simulink model "SC228_TrackedRadarModelUnitTest"  (R2018b)
settings: Solver=VariableStepAuto  StartTime=0.0  StopTime=180  RelTol=1e-3
model workspace (MAT data in the model file):
  MCOS : class17 (value not decoded)
  MCOS : class17 (value not decoded)
  MCOS : class17 (value not decoded)
  MCOS : class17 (value not decoded)
  MCOS : class17 (value not decoded)
  MCOS : class17 (value not decoded)
  N_tracked_random_stddev_ft = 250
  MCOS : class17 (value not decoded)
  MCOS : class17 (value not decoded)
  MCOS : class17 (value not decoded)
  MCOS : class17 (value not decoded)
  MCOS : class17 (value not decoded)
  MCOS : class17 (value not decoded)
  MCOS : class17 (value not decoded)
undefined symbols (not defined in the file or in its folder): ac1dyn_alt0_ft, ac1dyn_con, ac1dyn_lat0_rad, ac1dyn_lon0_rad, ac2dyn_alt0_ft, ac2dyn_con, ac2dyn_lat0_rad, ac2dyn_lon0_rad, ddh_ftps2, dh_ftps, dv_ftps2, e_ft, Edot_ftps, h_ft, hdot_ftps, latLonAltState, n_ft, Ndot_ftps, p_radps, phi_rad, phidot_radps, psi_rad, psidot_radps, q_radps, r_radps, theta_rad, thetadot_radps, uas_rdr_trckd_az_bias_ft, uas_rdr_trckd_az_bias_rad, uas_rdr_trckd_az_random_stddev_rad, uas_rdr_trckd_az_stddev_ft, uas_rdr_trckd_azdot_bias_ftps, uas_rdr_trckd_azdot_stddev_ftps, uas_rdr_trckd_debugMode, uas_rdr_trckd_dt_s, uas_rdr_trckd_el_bias_ft, uas_rdr_trckd_el_bias_rad, uas_rdr_trckd_el_random_stddev_rad, uas_rdr_trckd_el_stddev_ft, uas_rdr_trckd_eldot_bias_ftps, uas_rdr_trckd_eldot_stddev_ftps, uas_rdr_trckd_RCPR_Mode, uas_rdr_trckd_RCPR_Range_ft, uas_rdr_trckd_reported_errorCovRAE, uas_rdr_trckd_rng_bias_ft, uas_rdr_trckd_rng_random_stddev_ft, uas_rdr_trckd_rngdot_bias_ftps, uas_rdr_trckd_rngdot_random_stddev_ftps, uas_rdr_trckd_seed1, uas_rdr_trckd_seed2, uas_rdr_trckd_seed3, uas_rdr_trckd_seed4, uas_rdr_trckd_sns_for_azimuth_deg, uas_rdr_trckd_sns_for_elevation_deg, v_ftps, vdot_fpss
libraries: simulink x17, dspmtrx3 x1
(part 2 of 2)

== system SC228_TrackedRadarModelUnitTest/AC2 - Track Following/Follow Trajectory/Compute Euler Angles ==
  AircraftState : Inport
  Constraints : Inport  Port=2
  Bus Selector : BusSelector  OutputSignals=psi_rad,theta_rad,phi_rad
  Bus Selector1 : BusSelector  OutputSignals=dphi_radps_max
  Discrete Derivative : simulink/Discrete/Discrete Derivative  gainval=1.0  ICPrevScaledInput=0.0  OutMin=[]  OutMax=[]  OutDataType=fixdt(1, 16)  OutScaling=2^-10  DoSatur=off
  Discrete Derivative1 : simulink/Discrete/Discrete Derivative  gainval=1.0  ICPrevScaledInput=0.0  OutMin=[]  OutMax=[]  OutDataType=fixdt(1, 16)  OutScaling=2^-10  DoSatur=off
  Discrete Derivative2 : simulink/Discrete/Discrete Derivative  gainval=1.0  ICPrevScaledInput=0.0  OutMin=[]  OutMax=[]  OutDataType=fixdt(1, 16)  OutScaling=2^-10  DoSatur=off
  IC : InitialCondition  Value=0
  IC1 : InitialCondition  Value=0
  IC2 : InitialCondition  Value=0
  Saturation Dynamic : simulink/Discontinuities/Saturation Dynamic  OutMin=[]  OutMax=[]  OutDataTypeStr=Inherit: Same as second input  OutDataType=fixdt(1, 16)  OutScaling=2^-10  DoSatur=off
  Unary Minus : UnaryMinus
  Psi Dot : Outport
  Theta Dot : Outport  Port=2
  "Phi Dot " : Outport  Port=3
  wires:
  Constraints/1 -> Bus Selector1/1
  IC2/1 -> Saturation Dynamic/2
  IC1/1 -> Theta Dot/1
  IC/1 -> Psi Dot/1
  Discrete Derivative2/1 -> IC2/1
  Discrete Derivative1/1 -> IC1/1
  Discrete Derivative/1 -> IC/1
  Bus Selector/3 -> Discrete Derivative2/1  "<phi_rad>"
  Bus Selector/2 -> Discrete Derivative1/1  "<theta_rad>"
  Bus Selector/1 -> Discrete Derivative/1  "<psi_rad>"
  AircraftState/1 -> Bus Selector/1
  Saturation Dynamic/1 -> "Phi Dot "/1
  Bus Selector1/1 -> Unary Minus/1, Saturation Dynamic/1  "<dphi_radps_max>"
  Unary Minus/1 -> Saturation Dynamic/3

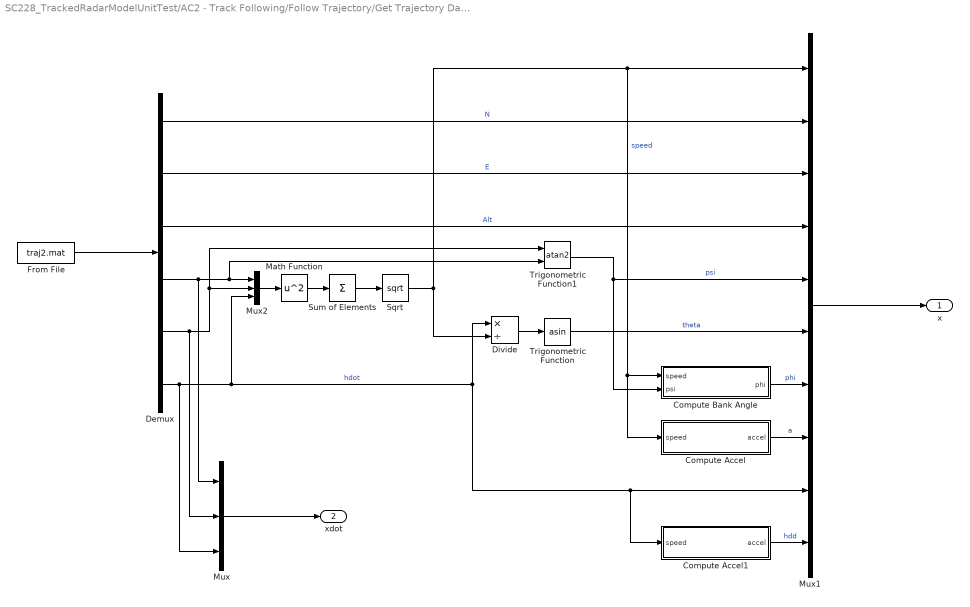
== system SC228_TrackedRadarModelUnitTest/AC2 - Track Following/Follow Trajectory/Get Trajectory Data ==
  Compute Accel : Subsystem
  Compute Accel1 : Subsystem
  Compute Bank Angle : Subsystem
  Demux : Demux  Outputs=6
  Divide : Product  Inputs=*/
  From File : FromFile  FileName=traj2.mat  SampleTime=0.1
  Math Function : Math  Operator=square  SaturateOnIntegerOverflow=on
  Mux : Mux  Inputs=3
  Mux1 : Mux  Inputs=10
  Mux2 : Mux  Inputs=3
  Sqrt : Sqrt  SaturateOnIntegerOverflow=on
  Sum of Elements : Sum  Inputs=+
  Trigonometric Function : Trigonometry  Operator=asin
  Trigonometric Function1 : Trigonometry  Operator=atan2
  x : Outport
  xdot : Outport  Port=2
  wires:
  Mux/1 -> xdot/1
  Compute Accel1/1(accel) -> Mux1/10  "hdd"
  Demux/5 -> Mux2/2, Trigonometric Function1/1, Mux/2
  Divide/1 -> Trigonometric Function/1
  Trigonometric Function1/1 -> Mux1/5, Compute Bank Angle/2(psi)  "psi"
  Trigonometric Function/1 -> Mux1/6  "theta"
  Compute Bank Angle/1(phi) -> Mux1/7  "phi"
  Compute Accel/1(accel) -> Mux1/8  "a"
  Mux1/1 -> x/1
  Sqrt/1 -> Divide/2, Mux1/1, Compute Bank Angle/1(speed), Compute Accel/1(speed)  "speed"
  Sum of Elements/1 -> Sqrt/1
  Math Function/1 -> Sum of Elements/1
  Mux2/1 -> Math Function/1
  Demux/6 -> Mux1/9, Compute Accel1/1(speed), Divide/1, Mux2/3, Mux/3  "hdot"
  Demux/4 -> Mux2/1, Trigonometric Function1/2, Mux/1
  Demux/3 -> Mux1/4  "Alt"
  Demux/2 -> Mux1/3  "E"
  Demux/1 -> Mux1/2  "N"
  From File/1 -> Demux/1

== system SC228_TrackedRadarModelUnitTest/AC2 - Track Following/Follow Trajectory/Null State Rate ==
  Bus Creator : BusCreator  Inputs='vdot_fpss','Ndot_ftps','Edot_ftps','hdot_ftps','psidot_radps','thetadot_radps','phidot_radps'  OutDataTypeStr=Bus: AircraftStateRate
  Constant{,1..6} (7 alike) : Constant  Value=0
  StateRate : Outport  OutDataTypeStr=Bus: AircraftStateRate
  wires:
  Constant6/1 -> Bus Creator/7  "phidot_radps"
  Constant5/1 -> Bus Creator/6  "thetadot_radps"
  Constant4/1 -> Bus Creator/5  "psidot_radps"
  Constant3/1 -> Bus Creator/4  "hdot_ftps"
  Constant2/1 -> Bus Creator/3  "Edot_ftps"
  Constant1/1 -> Bus Creator/2  "Ndot_ftps"
  Constant/1 -> Bus Creator/1  "vdot_fpss"
  Bus Creator/1 -> StateRate/1

== system SC228_TrackedRadarModelUnitTest/AC2 - Track Following/Follow Trajectory/Set LLA  ==
  State In : Inport
  Bus Assignment : BusAssignment  AssignedSignals=latLonAltState.lat_rad,latLonAltState.lon_rad,latLonAltState.dlat_radps,latLonAltState.dlon_radps,latLonAltState.alt_ft,latLonAltState.dalt_ftps
  Bus Selector : BusSelector  OutputSignals=e_ft,n_ft,h_ft,v_ftps,psi_rad,theta_rad
  Constant : Constant  Value=lat0
  Constant7 : Constant  Value=lon0
  Constant8 : Constant  Value=h0
  MATLAB Function : MATLAB Function  TreatAsAtomicUnit=on
  State Out : Outport
  wires:
  Bus Selector/6 -> MATLAB Function/6(theta_rad)  "<theta_rad>"
  Bus Selector/5 -> MATLAB Function/5(psi_rad)  "<psi_rad>"
  Bus Selector/4 -> MATLAB Function/4(v_ftps)  "<v_ftps>"
  Bus Selector/3 -> MATLAB Function/3(u_ft)  "<h_ft>"
  Bus Selector/2 -> MATLAB Function/2(n_ft)  "<n_ft>"
  Bus Selector/1 -> MATLAB Function/1(e_ft)  "<e_ft>"
  Constant8/1 -> MATLAB Function/9(h0)
  Constant7/1 -> MATLAB Function/8(lon0)
  Constant/1 -> MATLAB Function/7(lat0)
  State In/1 -> Bus Selector/1, Bus Assignment/1
  Bus Assignment/1 -> State Out/1
  MATLAB Function/6(dalt_ftps) -> Bus Assignment/7  "dalt_ftps"
  MATLAB Function/5(alt_ft) -> Bus Assignment/6  "alt_ft"
  MATLAB Function/4(dlon_radps) -> Bus Assignment/5  "dlon_radps"
  MATLAB Function/3(dlat_radps) -> Bus Assignment/4  "dlat_radps"
  MATLAB Function/2(lon_rad) -> Bus Assignment/3  "lon_rad"
  MATLAB Function/1(lat_rad) -> Bus Assignment/2  "lat_rad"

== system SC228_TrackedRadarModelUnitTest/AC2 - Track Following/Follow Trajectory/Set State ==
  x : Inport
  Bus Assignment : BusAssignment  AssignedSignals=v_ftps,n_ft,e_ft,h_ft,psi_rad,theta_rad,phi_rad,dv_ftps2,dh_ftps,ddh_ftps2
  Demux : Demux  Outputs=10
  Null AircraftState : Subsystem
  State : Outport
  wires:
  Demux/10 -> Bus Assignment/11
  Demux/9 -> Bus Assignment/10
  Bus Assignment/1 -> State/1
  Null AircraftState/1(State) -> Bus Assignment/1
  Demux/7 -> Bus Assignment/8  "phi"
  x/1 -> Demux/1
  Demux/6 -> Bus Assignment/7  "theta"
  Demux/5 -> Bus Assignment/6  "psi"
  Demux/4 -> Bus Assignment/5  "h"
  Demux/3 -> Bus Assignment/4  "E"
  Demux/2 -> Bus Assignment/3  "N"
  Demux/1 -> Bus Assignment/2  "v"
  Demux/8 -> Bus Assignment/9  "a"

== system SC228_TrackedRadarModelUnitTest/SC-228 Sensor Model: Radar (Tracked)/Add Errors/Colored Noise1 ==
  Add : Sum  Inputs=+++  SampleTime=dt
  Add1 : Sum  SampleTime=dt
  Constant : Constant  Value=false
  Constant1 : Constant  Value=0
  Gain : Gain  Gain=exp(-dt(1)/tau)  SampleTime=dt
  Gain1 : Gain  Gain=sig*sqrt(1-(exp(-dt(1)/tau))*(exp(-dt(1)/tau)))
  Gain2 : Gain  Gain=sig
  IsInitial : Memory  InitialCondition=true  InheritSampleTime=on
  Memory : Memory  InheritSampleTime=on
  Random Number : RandomNumber  Seed=seed  SampleTime=dt_s
  Switch : Switch  Criteria=u2 ~= 0  SampleTime=dt
  bias : Constant  Value=bias
  noisy : Outport
  wires:
  Gain2/1 -> Switch/1
  Add1/1 -> Switch/3  "colored random error"
  IsInitial/1 -> Switch/2
  Constant/1 -> IsInitial/1
  Memory/1 -> Gain/1
  Add/1 -> noisy/1  "noisy state parameter"
  Gain/1 -> Add1/1  "correlated error"
  Random Number/1 -> Gain1/1, Gain2/1
  bias/1 -> Add/2  "fixed bias"
  Switch/1 -> Add/3, Memory/1  "colored random error"
  Gain1/1 -> Add1/2  "uncorrelated error"
  Constant1/1 -> Add/1

== system SC228_TrackedRadarModelUnitTest/SC-228 Sensor Model: Radar (Tracked)/Add Errors/Colored Noise2 ==
  Add : Sum  Inputs=+++  SampleTime=dt
  Add1 : Sum  SampleTime=dt
  Constant : Constant  Value=false
  Constant1 : Constant  Value=0
  Gain : Gain  Gain=exp(-dt(1)/tau)  SampleTime=dt
  Gain1 : Gain  Gain=sig*sqrt(1-(exp(-dt(1)/tau))*(exp(-dt(1)/tau)))
  Gain2 : Gain  Gain=sig
  IsInitial : Memory  InitialCondition=true  InheritSampleTime=on
  Memory : Memory  InheritSampleTime=on
  Random Number : RandomNumber  Seed=seed  SampleTime=dt_s
  Switch : Switch  Criteria=u2 ~= 0  SampleTime=dt
  bias : Constant  Value=0
  noisy : Outport
  wires:
  Gain2/1 -> Switch/1
  Add1/1 -> Switch/3  "colored random error"
  IsInitial/1 -> Switch/2
  Constant/1 -> IsInitial/1
  Memory/1 -> Gain/1
  Add/1 -> noisy/1  "noisy state parameter"
  Gain/1 -> Add1/1  "correlated error"
  Random Number/1 -> Gain1/1, Gain2/1
  bias/1 -> Add/2  "fixed bias"
  Switch/1 -> Add/3, Memory/1  "colored random error"
  Gain1/1 -> Add1/2  "uncorrelated error"
  Constant1/1 -> Add/1

== system SC228_TrackedRadarModelUnitTest/SC-228 Sensor Model: Radar (Tracked)/Add Errors/Colored Noise3 ==
  Add : Sum  Inputs=+++  SampleTime=dt
  Add1 : Sum  SampleTime=dt
  Constant : Constant  Value=false
  Constant1 : Constant  Value=0
  Gain : Gain  Gain=exp(-dt(1)/tau)  SampleTime=dt
  Gain1 : Gain  Gain=sig*sqrt(1-(exp(-dt(1)/tau))*(exp(-dt(1)/tau)))
  Gain2 : Gain  Gain=sig
  IsInitial : Memory  InitialCondition=true  InheritSampleTime=on
  Memory : Memory  InheritSampleTime=on
  Random Number : RandomNumber  Seed=seed  SampleTime=dt_s
  Switch : Switch  Criteria=u2 ~= 0  SampleTime=dt
  bias : Constant  Value=0
  noisy : Outport
  wires:
  Gain2/1 -> Switch/1
  Add1/1 -> Switch/3  "colored random error"
  IsInitial/1 -> Switch/2
  Constant/1 -> IsInitial/1
  Memory/1 -> Gain/1
  Add/1 -> noisy/1  "noisy state parameter"
  Gain/1 -> Add1/1  "correlated error"
  Random Number/1 -> Gain1/1, Gain2/1
  bias/1 -> Add/2  "fixed bias"
  Switch/1 -> Add/3, Memory/1  "colored random error"
  Gain1/1 -> Add1/2  "uncorrelated error"
  Constant1/1 -> Add/1

== system SC228_TrackedRadarModelUnitTest/SC-228 Sensor Model: Radar (Tracked)/Add Errors/Colored Noise4 ==
  Add : Sum  Inputs=+++  SampleTime=dt
  Add1 : Sum  SampleTime=dt
  Constant : Constant  Value=false
  Constant1 : Constant  Value=0
  Gain : Gain  Gain=exp(-dt(1)/tau)  SampleTime=dt
  Gain1 : Gain  Gain=sig*sqrt(1-(exp(-dt(1)/tau))*(exp(-dt(1)/tau)))
  Gain2 : Gain  Gain=sig
  IsInitial : Memory  InitialCondition=true  InheritSampleTime=on
  Memory : Memory  InheritSampleTime=on
  Random Number : RandomNumber  Seed=seed  SampleTime=dt_s
  Switch : Switch  Criteria=u2 ~= 0  SampleTime=dt
  bias : Constant  Value=0
  noisy : Outport
  wires:
  Gain2/1 -> Switch/1
  Add1/1 -> Switch/3  "colored random error"
  IsInitial/1 -> Switch/2
  Constant/1 -> IsInitial/1
  Memory/1 -> Gain/1
  Add/1 -> noisy/1  "noisy state parameter"
  Gain/1 -> Add1/1  "correlated error"
  Random Number/1 -> Gain1/1, Gain2/1
  bias/1 -> Add/2  "fixed bias"
  Switch/1 -> Add/3, Memory/1  "colored random error"
  Gain1/1 -> Add1/2  "uncorrelated error"
  Constant1/1 -> Add/1

== system SC228_TrackedRadarModelUnitTest/SC-228 Sensor Model: Radar (Tracked)/Determine Validity/Determine if In Range ==
  prevIsValid : Inport
  rng_ft : Inport  Port=2
  intruderSpeed_ftps : Inport  Port=3
  azimuth_deg : Inport  Port=4
  Constant : Constant  Value=debugMode
  Constant1 : Constant  Value=RCPR_Mode
  Constant2 : Constant  Value=RCPR_Range_ft
  Convert to Knots : Gain  Gain=0.592484
  MATLAB Function : MATLAB Function  TreatAsAtomicUnit=on
  To Workspace : ToWorkspace  VariableName=maxRange_ft  SaveFormat=Timeseries  SampleTime=-1
  rangeValid : Outport
  wires:
  Constant2/1 -> MATLAB Function/7(RCPR_Range_ft)
  Constant1/1 -> MATLAB Function/6(RCPR_Mode)
  rng_ft/1 -> MATLAB Function/1(range)
  MATLAB Function/1(rangeValid) -> rangeValid/1
  intruderSpeed_ftps/1 -> Convert to Knots/1
  prevIsValid/1 -> MATLAB Function/4(prevIsValid)
  Convert to Knots/1 -> MATLAB Function/3(intruderSpeed)
  azimuth_deg/1 -> MATLAB Function/2(azimuth)
  Constant/1 -> MATLAB Function/5(debugMode)
  MATLAB Function/2(maxRange) -> To Workspace/1

== system SC228_TrackedRadarModelUnitTest/AC1 - Track Following/Follow Trajectory/Compute Body Rates/Compute p ==
  State : Inport
  Euler Rates : Inport  Port=2
  Add : Sum
  Bus Selector : BusSelector  OutputSignals=theta_rad
  Bus Selector1 : BusSelector  OutputSignals=psidot,phidot
  Product : Product
  Trigonometric Function : Trigonometry
  Unary Minus : UnaryMinus
  p : Outport
  wires:
  Add/1 -> p/1
  Unary Minus/1 -> Product/1
  Bus Selector1/2 -> Add/2  "<phidot>"
  Product/1 -> Add/1
  Trigonometric Function/1 -> Unary Minus/1
  State/1 -> Bus Selector/1
  Euler Rates/1 -> Bus Selector1/1
  Bus Selector/1 -> Trigonometric Function/1  "<theta_rad>"
  Bus Selector1/1 -> Product/2  "<psidot>"

== system SC228_TrackedRadarModelUnitTest/AC1 - Track Following/Follow Trajectory/Compute Body Rates/Compute q ==
  State : Inport
  Euler Rates : Inport  Port=2
  Add : Sum
  Bus Selector : BusSelector  OutputSignals=phi_rad,theta_rad
  Bus Selector1 : BusSelector  OutputSignals=thetadot,psidot
  Product : Product
  Product1 : Product  Inputs=3
  Trigonometric Function : Trigonometry  Operator=cos
  Trigonometric Function1 : Trigonometry  Operator=cos
  Trigonometric Function2 : Trigonometry
  q : Outport
  wires:
  Add/1 -> q/1
  Product1/1 -> Add/2
  Bus Selector1/2 -> Product1/3  "<psidot>"
  Trigonometric Function1/1 -> Product1/2
  Trigonometric Function2/1 -> Product1/1
  Bus Selector/2 -> Trigonometric Function1/1  "<theta_rad>"
  Bus Selector1/1 -> Product/2  "<thetadot>"
  Bus Selector/1 -> Trigonometric Function/1, Trigonometric Function2/1  "<phi_rad>"
  Trigonometric Function/1 -> Product/1
  Product/1 -> Add/1
  State/1 -> Bus Selector/1
  Euler Rates/1 -> Bus Selector1/1

== system SC228_TrackedRadarModelUnitTest/AC1 - Track Following/Follow Trajectory/Compute Body Rates/Compute r ==
  State : Inport
  Euler Rates : Inport  Port=2
  Add : Sum
  Bus Selector : BusSelector  OutputSignals=phi_rad,theta_rad
  Bus Selector1 : BusSelector  OutputSignals=thetadot,psidot
  Product : Product
  Product1 : Product  Inputs=3
  Trigonometric Function : Trigonometry
  Trigonometric Function1 : Trigonometry  Operator=cos
  Trigonometric Function2 : Trigonometry  Operator=cos
  Unary Minus : UnaryMinus
  r : Outport
  wires:
  Unary Minus/1 -> Product/1
  Add/1 -> r/1
  Product1/1 -> Add/2
  Bus Selector1/2 -> Product1/3  "<psidot>"
  Trigonometric Function1/1 -> Product1/2
  Trigonometric Function2/1 -> Product1/1
  Bus Selector/2 -> Trigonometric Function1/1  "<theta_rad>"
  Bus Selector1/1 -> Product/2  "<thetadot>"
  Bus Selector/1 -> Trigonometric Function/1, Trigonometric Function2/1  "<phi_rad>"
  Trigonometric Function/1 -> Unary Minus/1
  Product/1 -> Add/1
  State/1 -> Bus Selector/1
  Euler Rates/1 -> Bus Selector1/1

== system SC228_TrackedRadarModelUnitTest/AC1 - Track Following/Follow Trajectory/Get Trajectory Data/Compute Accel ==
  speed : Inport
  Discrete Derivative : simulink/Discrete/Discrete Derivative  gainval=1.0  ICPrevScaledInput=0.0  OutMin=[]  OutMax=[]  OutDataType=fixdt(1, 16)  OutScaling=2^-10  DoSatur=off
  accel : Outport
  wires:
  Discrete Derivative/1 -> accel/1
  speed/1 -> Discrete Derivative/1

== system SC228_TrackedRadarModelUnitTest/AC1 - Track Following/Follow Trajectory/Get Trajectory Data/Compute Accel1 ==
  speed : Inport
  Discrete Derivative : simulink/Discrete/Discrete Derivative  gainval=1.0  ICPrevScaledInput=0.0  OutMin=[]  OutMax=[]  OutDataType=fixdt(1, 16)  OutScaling=2^-10  DoSatur=off
  accel : Outport
  wires:
  Discrete Derivative/1 -> accel/1
  speed/1 -> Discrete Derivative/1

== system SC228_TrackedRadarModelUnitTest/AC1 - Track Following/Follow Trajectory/Get Trajectory Data/Compute Bank Angle ==
  speed : Inport
  psi : Inport  Port=2
  Constant : Constant  Value=32.2
  Discrete Derivative : simulink/Discrete/Discrete Derivative  gainval=1.0  ICPrevScaledInput=0.0  OutMin=[]  OutMax=[]  OutDataType=fixdt(1, 16)  OutScaling=2^-10  DoSatur=off
  Divide : Product  Inputs=*/
  IC : InitialCondition  Value=0
  Product : Product
  Trigonometric Function : Trigonometry  Operator=atan
  phi : Outport
  wires:
  IC/1 -> Product/2
  Trigonometric Function/1 -> phi/1
  Divide/1 -> Trigonometric Function/1
  Constant/1 -> Divide/2
  Product/1 -> Divide/1
  psi/1 -> Discrete Derivative/1  "psi"
  speed/1 -> Product/1  "speed"
  Discrete Derivative/1 -> IC/1  "psidot"

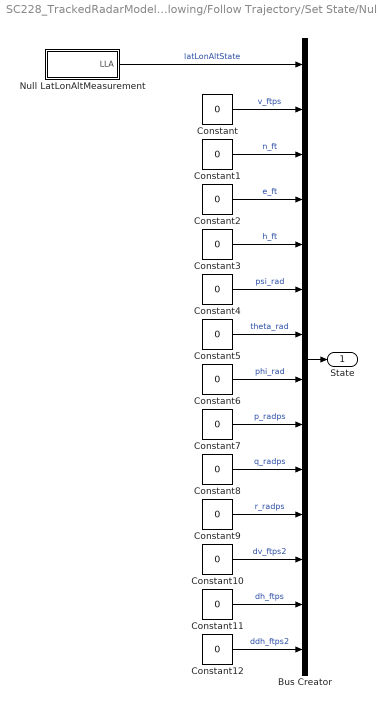
== system SC228_TrackedRadarModelUnitTest/AC1 - Track Following/Follow Trajectory/Set State/Null AircraftState ==
  Bus Creator : BusCreator  Inputs='latLonAltState','v_ftps','n_ft','e_ft','h_ft','psi_rad','theta_rad','phi_rad','p_radps','q_radps','r_radps','dv_ftps2','dh_ftps','ddh_ftps2'  OutDataTypeStr=Bus: AircraftState
  Constant{,1..12} (13 alike) : Constant  Value=0
  Null LatLonAltMeasurement : Subsystem
  State : Outport
  wires:
  Null LatLonAltMeasurement/1(LLA) -> Bus Creator/1  "latLonAltState"
  Constant/1 -> Bus Creator/2  "v_ftps"
  Constant12/1 -> Bus Creator/14  "ddh_ftps2"
  Constant1/1 -> Bus Creator/3  "n_ft"
  Bus Creator/1 -> State/1
  Constant6/1 -> Bus Creator/8  "phi_rad"
  Constant10/1 -> Bus Creator/12  "dv_ftps2"
  Constant7/1 -> Bus Creator/9  "p_radps"
  Constant5/1 -> Bus Creator/7  "theta_rad"
  Constant4/1 -> Bus Creator/6  "psi_rad"
  Constant8/1 -> Bus Creator/10  "q_radps"
  Constant9/1 -> Bus Creator/11  "r_radps"
  Constant3/1 -> Bus Creator/5  "h_ft"
  Constant2/1 -> Bus Creator/4  "e_ft"
  Constant11/1 -> Bus Creator/13  "dh_ftps"

== system SC228_TrackedRadarModelUnitTest/AC2 - Track Following/Follow Trajectory/Compute Body Rates/Compute p ==
  State : Inport
  Euler Rates : Inport  Port=2
  Add : Sum
  Bus Selector : BusSelector  OutputSignals=theta_rad
  Bus Selector1 : BusSelector  OutputSignals=psidot,phidot
  Product : Product
  Trigonometric Function : Trigonometry
  Unary Minus : UnaryMinus
  p : Outport
  wires:
  Add/1 -> p/1
  Unary Minus/1 -> Product/1
  Bus Selector1/2 -> Add/2  "<phidot>"
  Product/1 -> Add/1
  Trigonometric Function/1 -> Unary Minus/1
  State/1 -> Bus Selector/1
  Euler Rates/1 -> Bus Selector1/1
  Bus Selector/1 -> Trigonometric Function/1  "<theta_rad>"
  Bus Selector1/1 -> Product/2  "<psidot>"

== system SC228_TrackedRadarModelUnitTest/AC2 - Track Following/Follow Trajectory/Compute Body Rates/Compute q ==
  State : Inport
  Euler Rates : Inport  Port=2
  Add : Sum
  Bus Selector : BusSelector  OutputSignals=phi_rad,theta_rad
  Bus Selector1 : BusSelector  OutputSignals=thetadot,psidot
  Product : Product
  Product1 : Product  Inputs=3
  Trigonometric Function : Trigonometry  Operator=cos
  Trigonometric Function1 : Trigonometry  Operator=cos
  Trigonometric Function2 : Trigonometry
  q : Outport
  wires:
  Add/1 -> q/1
  Product1/1 -> Add/2
  Bus Selector1/2 -> Product1/3  "<psidot>"
  Trigonometric Function1/1 -> Product1/2
  Trigonometric Function2/1 -> Product1/1
  Bus Selector/2 -> Trigonometric Function1/1  "<theta_rad>"
  Bus Selector1/1 -> Product/2  "<thetadot>"
  Bus Selector/1 -> Trigonometric Function/1, Trigonometric Function2/1  "<phi_rad>"
  Trigonometric Function/1 -> Product/1
  Product/1 -> Add/1
  State/1 -> Bus Selector/1
  Euler Rates/1 -> Bus Selector1/1

== system SC228_TrackedRadarModelUnitTest/AC2 - Track Following/Follow Trajectory/Compute Body Rates/Compute r ==
  State : Inport
  Euler Rates : Inport  Port=2
  Add : Sum
  Bus Selector : BusSelector  OutputSignals=phi_rad,theta_rad
  Bus Selector1 : BusSelector  OutputSignals=thetadot,psidot
  Product : Product
  Product1 : Product  Inputs=3
  Trigonometric Function : Trigonometry
  Trigonometric Function1 : Trigonometry  Operator=cos
  Trigonometric Function2 : Trigonometry  Operator=cos
  Unary Minus : UnaryMinus
  r : Outport
  wires:
  Unary Minus/1 -> Product/1
  Add/1 -> r/1
  Product1/1 -> Add/2
  Bus Selector1/2 -> Product1/3  "<psidot>"
  Trigonometric Function1/1 -> Product1/2
  Trigonometric Function2/1 -> Product1/1
  Bus Selector/2 -> Trigonometric Function1/1  "<theta_rad>"
  Bus Selector1/1 -> Product/2  "<thetadot>"
  Bus Selector/1 -> Trigonometric Function/1, Trigonometric Function2/1  "<phi_rad>"
  Trigonometric Function/1 -> Unary Minus/1
  Product/1 -> Add/1
  State/1 -> Bus Selector/1
  Euler Rates/1 -> Bus Selector1/1

== system SC228_TrackedRadarModelUnitTest/AC2 - Track Following/Follow Trajectory/Get Trajectory Data/Compute Accel ==
  speed : Inport
  Discrete Derivative : simulink/Discrete/Discrete Derivative  gainval=1.0  ICPrevScaledInput=0.0  OutMin=[]  OutMax=[]  OutDataType=fixdt(1, 16)  OutScaling=2^-10  DoSatur=off
  accel : Outport
  wires:
  Discrete Derivative/1 -> accel/1
  speed/1 -> Discrete Derivative/1

== system SC228_TrackedRadarModelUnitTest/AC2 - Track Following/Follow Trajectory/Get Trajectory Data/Compute Accel1 ==
  speed : Inport
  Discrete Derivative : simulink/Discrete/Discrete Derivative  gainval=1.0  ICPrevScaledInput=0.0  OutMin=[]  OutMax=[]  OutDataType=fixdt(1, 16)  OutScaling=2^-10  DoSatur=off
  accel : Outport
  wires:
  Discrete Derivative/1 -> accel/1
  speed/1 -> Discrete Derivative/1

== system SC228_TrackedRadarModelUnitTest/AC2 - Track Following/Follow Trajectory/Get Trajectory Data/Compute Bank Angle ==
  speed : Inport
  psi : Inport  Port=2
  Constant : Constant  Value=32.2
  Discrete Derivative : simulink/Discrete/Discrete Derivative  gainval=1.0  ICPrevScaledInput=0.0  OutMin=[]  OutMax=[]  OutDataType=fixdt(1, 16)  OutScaling=2^-10  DoSatur=off
  Divide : Product  Inputs=*/
  IC : InitialCondition  Value=0
  Product : Product
  Trigonometric Function : Trigonometry  Operator=atan
  phi : Outport
  wires:
  IC/1 -> Product/2
  Trigonometric Function/1 -> phi/1
  Divide/1 -> Trigonometric Function/1
  Constant/1 -> Divide/2
  Product/1 -> Divide/1
  psi/1 -> Discrete Derivative/1  "psi"
  speed/1 -> Product/1  "speed"
  Discrete Derivative/1 -> IC/1  "psidot"

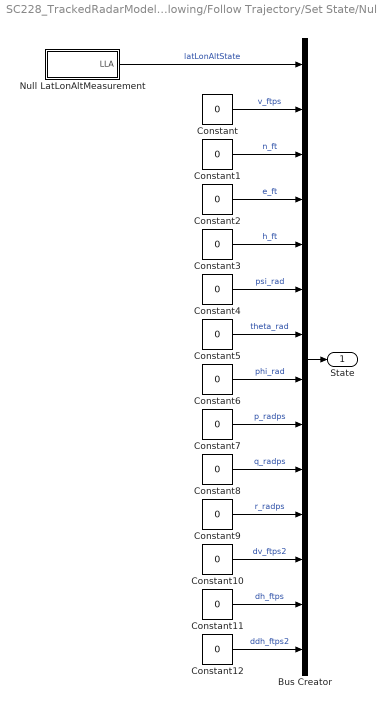
== system SC228_TrackedRadarModelUnitTest/AC2 - Track Following/Follow Trajectory/Set State/Null AircraftState ==
  Bus Creator : BusCreator  Inputs='latLonAltState','v_ftps','n_ft','e_ft','h_ft','psi_rad','theta_rad','phi_rad','p_radps','q_radps','r_radps','dv_ftps2','dh_ftps','ddh_ftps2'  OutDataTypeStr=Bus: AircraftState
  Constant{,1..12} (13 alike) : Constant  Value=0
  Null LatLonAltMeasurement : Subsystem
  State : Outport
  wires:
  Null LatLonAltMeasurement/1(LLA) -> Bus Creator/1  "latLonAltState"
  Constant/1 -> Bus Creator/2  "v_ftps"
  Constant12/1 -> Bus Creator/14  "ddh_ftps2"
  Constant1/1 -> Bus Creator/3  "n_ft"
  Bus Creator/1 -> State/1
  Constant6/1 -> Bus Creator/8  "phi_rad"
  Constant10/1 -> Bus Creator/12  "dv_ftps2"
  Constant7/1 -> Bus Creator/9  "p_radps"
  Constant5/1 -> Bus Creator/7  "theta_rad"
  Constant4/1 -> Bus Creator/6  "psi_rad"
  Constant8/1 -> Bus Creator/10  "q_radps"
  Constant9/1 -> Bus Creator/11  "r_radps"
  Constant3/1 -> Bus Creator/5  "h_ft"
  Constant2/1 -> Bus Creator/4  "e_ft"
  Constant11/1 -> Bus Creator/13  "dh_ftps"

== system SC228_TrackedRadarModelUnitTest/AC1 - Track Following/Follow Trajectory/Set State/Null AircraftState/Null LatLonAltMeasurement ==
  Bus Creator : BusCreator  Inputs='lat_rad','lon_rad','dlat_radps','dlon_radps','alt_ft','dalt_ftps'  OutDataTypeStr=Bus: LatLonAltMeasurement
  Constant{,1..5} (6 alike) : Constant  Value=0
  LLA : Outport
  wires:
  Constant1/1 -> Bus Creator/2  "lon_rad"
  Bus Creator/1 -> LLA/1
  Constant4/1 -> Bus Creator/5  "alt_ft"
  Constant5/1 -> Bus Creator/6  "dalt_ftps"
  Constant3/1 -> Bus Creator/4  "dlon_radps"
  Constant/1 -> Bus Creator/1  "lat_rad"
  Constant2/1 -> Bus Creator/3  "dlat_radps"

== system SC228_TrackedRadarModelUnitTest/AC2 - Track Following/Follow Trajectory/Set State/Null AircraftState/Null LatLonAltMeasurement ==
  Bus Creator : BusCreator  Inputs='lat_rad','lon_rad','dlat_radps','dlon_radps','alt_ft','dalt_ftps'  OutDataTypeStr=Bus: LatLonAltMeasurement
  Constant{,1..5} (6 alike) : Constant  Value=0
  LLA : Outport
  wires:
  Constant1/1 -> Bus Creator/2  "lon_rad"
  Bus Creator/1 -> LLA/1
  Constant4/1 -> Bus Creator/5  "alt_ft"
  Constant5/1 -> Bus Creator/6  "dalt_ftps"
  Constant3/1 -> Bus Creator/4  "dlon_radps"
  Constant/1 -> Bus Creator/1  "lat_rad"
  Constant2/1 -> Bus Creator/3  "dlat_radps"

== matlab function SC228_TrackedRadarModelUnitTest/AC1 - Track Following/Follow Trajectory/Set LLA /MATLAB Function ==
  data: e_ft input; n_ft input; u_ft input; v_ftps input; psi_rad input; theta_rad input; lat0 input; lat_rad output; lon0 input; h0 input; lon_rad output; dlat_radps output; dlon_radps output; alt_ft output; dalt_ftps output
function [lat_rad,lon_rad,dlat_radps,dlon_radps,alt_ft,dalt_ftps] = convertToLLA(e_ft,n_ft,u_ft,v_ftps,psi_rad,theta_rad,lat0,lon0,h0)
%#codegen

% WGS-84 ellipsoid constants
a = 2.09256*10^7;          %Semi-major axis (meters)
f = 1.0/298.257223563;  %Flattening
ecc_sq = f*(2.0-f);        %Eccentricity^2


% Ellipsoidal "radius"
er = a./sqrt(1-ecc_sq.*sin(lat0).^2);


% ECEF coordinates
x0 = (er + h0)*cos(lat0)*cos(lon0);
y0 = (er + h0)*cos(lat0)*sin(lon0);
z0 = (er.*(1-ecc_sq) + h0)*sin(lat0);


%% Rotation Matrix
posECEF0 = [x0;y0;z0];
% Compute the local Up unit vector
vHatU = posECEF0;
vHatU(3) = vHatU(3) ./ ((1-f)^2);
vHatU = vHatU ./ norm(vHatU);

% Compute the projection onto the local Up vector
pU = vHatU * vHatU';

% Compute the projection onto the local Tangent plane
pT = eye(size(pU)) - pU;

% Compute the local North unit vector
vHatZ = [0;0;1];
vHatN = pT * vHatZ;
vHatN = vHatN ./ norm(vHatN);

% Compute the local East unit vector
vHatE = cross(vHatN,vHatU);

% Compute ENU rotation matrix
rotMatENU = zeros(3,3);
rotMatENU(:,1) = vHatE;
rotMatENU(:,2) = vHatN;
rotMatENU(:,3) = vHatU;

tPosECEF = rotMatENU*[e_ft;n_ft;u_ft] + [x0;y0;z0];


%% ECEF to LLA
% WGS-84 derived parameters
b = (1-f).*a;                       %Semi-minor axis (meters)
ecc1_sq = (a.^2 - b.^2)./(a.^2);    %First eccentricity squared
ecc2_sq = (a.^2 - b.^2)./(b.^2);    %Second eccentricity squared


% Length of position vector in equatorial plane
rho = sqrt(tPosECEF(1).^2 + tPosECEF(2).^2);

% Auxillary angle
theta = atan( (tPosECEF(3).*a)./(rho.*b) );

lon_rad = atan2(tPosECEF(2),tPosECEF(1));
lat_rad = atan( (tPosECEF(3) + ecc2_sq.*b.*(sin(theta)).^3)./(rho - ecc1_sq.*a.*(cos(theta)).^3) );

ewRadCurv = a./sqrt(1-ecc1_sq.*sin(lat_rad).^2);

alt_ft = (rho./cos(lat_rad)) - ewRadCurv;


%% Velocities - Project 1 sec into future and use to estimate
dalt_ftps = v_ftps*sin(theta_rad); % Assume about the same


tPosECEF_1sec = rotMatENU*[e_ft+v_ftps*sin(theta_rad)*sin(psi_rad);...
                           n_ft+v_ftps*sin(theta_rad)*cos(psi_rad);...
                           u_ft] + ...
                           [x0;y0;z0];

% Length of position vector in equatorial plane
rho = sqrt(tPosECEF_1sec(1).^2 + tPosECEF_1sec(2).^2);

% Auxillary angle
theta = atan( (tPosECEF_1sec(3).*a)./(rho.*b) );

lon_rad_1sec = atan2(tPosECEF_1sec(2),tPosECEF_1sec(1));
lat_rad_1sec = atan( (tPosECEF_1sec(3) + ecc2_sq.*b.*(sin(theta)).^3)./(rho - ecc1_sq.*a.*(cos(theta)).^3) );

dlat_radps = lat_rad_1sec - lat_rad;
dlon_radps = lon_rad_1sec - lon_rad;
end

== matlab function SC228_TrackedRadarModelUnitTest/NED2FRD ==
  data: psi_rad input; T output; theta input; phi input
function T = Transform_NED2FRD(psi_rad,theta,phi)
%#codegen

yaw = [ cos(psi_rad) sin(psi_rad) 0;
       -sin(psi_rad) cos(psi_rad) 0;
               0        0 1 ];
           
pitch = [ cos(theta) 0 -sin(theta);
                   0 1           0;
          sin(theta) 0  cos(theta) ];
      
roll = [ 1         0        0;
         0  cos(phi) sin(phi);
         0 -sin(phi) cos(phi) ];
     
T = roll*pitch*yaw;     % transformation FROM geographic coord TO body coord

== matlab function SC228_TrackedRadarModelUnitTest/sph2cart ==
  data: x output; r input; az_rad input; el_rad input; y output; z_d output; xdot output; ydot output; zdot output; J output; rdot input; azdot_radps input; eldot_radps input; K output
function [x,y,z_d, xdot,ydot,zdot, J, K] = spherical2cartesian(r,az_rad,el_rad, rdot, azdot_radps, eldot_radps)
%Convert Range, Azimuth, Elevation to North, East, Down coordinates
% Returns the Jacobian J of the 3x3 transformation and the off-diagonal
% Jacobian block K for the 6x6 transformation (so J' = [J zeros(3); K J])

x = r*cos(el_rad)*cos(az_rad);
y = r*cos(el_rad)*sin(az_rad);
z_d = -r*sin(el_rad);

% Jacobian (x,y,z)/(r,az,el)
J = [  x/r  -y   z_d*cos(az_rad); ...
       y/r   x   z_d*sin(az_rad); ...
       z_d/r   0  -r*cos(el_rad) ];
   
% d(x,y,z)/dt = J * d(r,az,el)/dt
xdot = J(1,:)*[rdot; azdot_radps; eldot_radps];
ydot = J(2,:)*[rdot; azdot_radps; eldot_radps];
zdot = J(3,:)*[rdot; azdot_radps; eldot_radps];
   
% position-velocity correlations
Kxdot_r = -(y/r)*azdot_radps + (z_d/r)*cos(az_rad)*eldot_radps;
Kxdot_az = -rdot*(y/r) - x*azdot_radps - z_d*sin(az_rad)*eldot_radps;
Kxdot_el = rdot*(z_d/r)*cos(az_rad) - z_d*sin(az_rad)*azdot_radps - x*eldot_radps;

Kydot_r = (z_d/r)*sin(az_rad)*eldot_radps + (x/r)*azdot_radps;
Kydot_az = rdot*(x/r) + z_d*cos(az_rad)*eldot_radps - y*azdot_radps;
Kydot_el = rdot*(z_d/r)*sin(az_rad) - y*eldot_radps + z_d*cos(az_rad)*azdot_radps;

Kzdot_r = -cos(el_rad)*eldot_radps;
Kzdot_az = 0;
Kzdot_el = -rdot*cos(el_rad) - z_d*eldot_radps;

K = [ Kxdot_r   Kxdot_az   Kxdot_el;
      Kydot_r   Kydot_az   Kydot_el;
      Kzdot_r   Kzdot_az   Kzdot_el   ];

== matlab function SC228_TrackedRadarModelUnitTest/AC2 - Track Following/Follow Trajectory/Set LLA /MATLAB Function ==
  data: e_ft input; n_ft input; u_ft input; v_ftps input; psi_rad input; theta_rad input; lat0 input; lat_rad output; lon0 input; h0 input; lon_rad output; dlat_radps output; dlon_radps output; alt_ft output; dalt_ftps output
function [lat_rad,lon_rad,dlat_radps,dlon_radps,alt_ft,dalt_ftps] = convertToLLA(e_ft,n_ft,u_ft,v_ftps,psi_rad,theta_rad,lat0,lon0,h0)
%#codegen

% WGS-84 ellipsoid constants
a = 2.09256*10^7;          %Semi-major axis (meters)
f = 1.0/298.257223563;  %Flattening
ecc_sq = f*(2.0-f);        %Eccentricity^2


% Ellipsoidal "radius"
er = a./sqrt(1-ecc_sq.*sin(lat0).^2);


% ECEF coordinates
x0 = (er + h0)*cos(lat0)*cos(lon0);
y0 = (er + h0)*cos(lat0)*sin(lon0);
z0 = (er.*(1-ecc_sq) + h0)*sin(lat0);


%% Rotation Matrix
posECEF0 = [x0;y0;z0];
% Compute the local Up unit vector
vHatU = posECEF0;
vHatU(3) = vHatU(3) ./ ((1-f)^2);
vHatU = vHatU ./ norm(vHatU);

% Compute the projection onto the local Up vector
pU = vHatU * vHatU';

% Compute the projection onto the local Tangent plane
pT = eye(size(pU)) - pU;

% Compute the local North unit vector
vHatZ = [0;0;1];
vHatN = pT * vHatZ;
vHatN = vHatN ./ norm(vHatN);

% Compute the local East unit vector
vHatE = cross(vHatN,vHatU);

% Compute ENU rotation matrix
rotMatENU = zeros(3,3);
rotMatENU(:,1) = vHatE;
rotMatENU(:,2) = vHatN;
rotMatENU(:,3) = vHatU;

tPosECEF = rotMatENU*[e_ft;n_ft;u_ft] + [x0;y0;z0];


%% ECEF to LLA
% WGS-84 derived parameters
b = (1-f).*a;                       %Semi-minor axis (meters)
ecc1_sq = (a.^2 - b.^2)./(a.^2);    %First eccentricity squared
ecc2_sq = (a.^2 - b.^2)./(b.^2);    %Second eccentricity squared


% Length of position vector in equatorial plane
rho = sqrt(tPosECEF(1).^2 + tPosECEF(2).^2);

% Auxillary angle
theta = atan( (tPosECEF(3).*a)./(rho.*b) );

lon_rad = atan2(tPosECEF(2),tPosECEF(1));
lat_rad = atan( (tPosECEF(3) + ecc2_sq.*b.*(sin(theta)).^3)./(rho - ecc1_sq.*a.*(cos(theta)).^3) );

ewRadCurv = a./sqrt(1-ecc1_sq.*sin(lat_rad).^2);

alt_ft = (rho./cos(lat_rad)) - ewRadCurv;


%% Velocities - Project 1 sec into future and use to estimate
dalt_ftps = v_ftps*sin(theta_rad); % Assume about the same


tPosECEF_1sec = rotMatENU*[e_ft+v_ftps*sin(theta_rad)*sin(psi_rad);...
                           n_ft+v_ftps*sin(theta_rad)*cos(psi_rad);...
                           u_ft] + ...
                           [x0;y0;z0];

% Length of position vector in equatorial plane
rho = sqrt(tPosECEF_1sec(1).^2 + tPosECEF_1sec(2).^2);

% Auxillary angle
theta = atan( (tPosECEF_1sec(3).*a)./(rho.*b) );

lon_rad_1sec = atan2(tPosECEF_1sec(2),tPosECEF_1sec(1));
lat_rad_1sec = atan( (tPosECEF_1sec(3) + ecc2_sq.*b.*(sin(theta)).^3)./(rho - ecc1_sq.*a.*(cos(theta)).^3) );

dlat_radps = lat_rad_1sec - lat_rad;
dlon_radps = lon_rad_1sec - lon_rad;
end

== matlab function SC228_TrackedRadarModelUnitTest/SC-228 Sensor Model: Radar (Tracked)/Add Errors/cart2sph ==
  data: x input; r output; az_rad output; el_rad output; rdot output; azdot_radps output; eldot_radps output; y input; z_d input; J output; xdot input; ydot input; zdot input; K output
function [r,az_rad,el_rad,rdot,azdot_radps,eldot_radps,J,K] = cartesian2spherical(x, y, z_d, xdot, ydot, zdot)
%Convert North, East, Down coordinates to Range, Azimuth, Elevation
% Returns the Jacobian J of the 3x3 transformation and the off-diagonal
% Jacobian block K for the 6x6 transformation (so J' = [J zeros(3); K J])

% range
xyz = [ x; y; z_d ];
r = norm(xyz);

% azimuth and azimuth rate
az_rad = atan2(y,x);

% elevation and elevation rate
el_rad = asin(-z_d/r);

% Jacobian (r,az,el)/(x,y,z)
h = norm( [ x y ] );
J = [       xyz'/r; ...
      -y/h^2      x/h^2        0; ...
      x*z_d/(h*r^2) y*z_d/(h*r^2) -h/r^2 ];

% d(r,za,el)/dt = J * d(x,y,z)/dt
rdot = J(1,:) * [xdot; ydot; zdot];
azdot_radps = J(2,:) * [xdot; ydot; zdot];
eldot_radps = J(3,:) * [xdot; ydot; zdot];
  
% position-velocity correlations (copied from sph->cart, get inverse of that K with Schur complement)
Kxdot_r = -(y/r)*azdot_radps + (z_d/r)*cos(az_rad)*eldot_radps;
Kxdot_az = -rdot*(y/r) - x*azdot_radps - z_d*sin(az_rad)*eldot_radps;
Kxdot_el = rdot*(z_d/r)*cos(az_rad) - z_d*sin(az_rad)*azdot_radps - x*eldot_radps;

Kydot_r = (z_d/r)*sin(az_rad)*eldot_radps + (x/r)*azdot_radps;
Kydot_az = rdot*(x/r) + z_d*cos(az_rad)*eldot_radps - y*azdot_radps;
Kydot_el = rdot*(z_d/r)*sin(az_rad) - y*eldot_radps + z_d*cos(az_rad)*azdot_radps;

Kzdot_r = -cos(el_rad)*eldot_radps;
Kzdot_az = 0;
Kzdot_el = -rdot*cos(el_rad) - z_d*eldot_radps;

K = -J*[ Kxdot_r   Kxdot_az   Kxdot_el;
         Kydot_r   Kydot_az   Kydot_el;
         Kzdot_r   Kzdot_az   Kzdot_el   ]*J;

== matlab function SC228_TrackedRadarModelUnitTest/SC-228 Sensor Model: Radar (Tracked)/Determine Validity/Determine if In Range/MATLAB Function ==
  data: range input; azimuth input; intruderSpeed input; rangeValid output; prevIsValid input; debugMode input; maxRange output; RCPR_Mode input; RCPR_Range_ft input
function [rangeValid, maxRange] = determineRangeValidity(range, azimuth, intruderSpeed, prevIsValid, debugMode, RCPR_Mode, RCPR_Range_ft)
%#codegen
maxRange = 0;

if(debugMode)
    if(RCPR_Mode)
        rangeValid = range >= RCPR_Range_ft;
    else
        rangeValid = true; 
    end
    maxRange = Inf;
    return;
end

azimuth = abs(azimuth);

if(intruderSpeed<100)
    DR = 5.4*6070;
    %Do not perform scale factor correction once track is established
    %DR scale factor is linearly interpolated between levels
    if(azimuth<=30)
        maxRange = DR*(1-0.33*(azimuth-0)/(30-0)*~prevIsValid);
    elseif(azimuth<=60)
        maxRange = DR*(1-(0.33+0.22*(azimuth-30)/(60-30))*~prevIsValid);   
    elseif(azimuth<=90)
        maxRange = DR*(1-(0.55+0.1*(azimuth-60)/(90-60))*~prevIsValid);   
    elseif(azimuth<=110)
        maxRange = DR*(1-(0.65+0.0*(azimuth-90)/(110-90))*~prevIsValid);   
    end
    
elseif (intruderSpeed>=100 && intruderSpeed<=130)
    DR = 6.0*6070;
    %Do not perform scale factor correction once track is established
    %DR scale factor is linearly interpolated between levels
    if(azimuth<=30)
        maxRange = DR*(1-0.22*(azimuth-0)/(30-0)*~prevIsValid);
    elseif(azimuth<=60)
        maxRange = DR*(1-(0.22+0.26*(azimuth-30)/(60-30))*~prevIsValid);   
    elseif(azimuth<=90)
        maxRange = DR*(1-(0.48+0.09*(azimuth-60)/(90-60))*~prevIsValid);   
    elseif(azimuth<=110)
        maxRange = DR*(1-(0.57+0.0*(azimuth-90)/(110-90))*~prevIsValid);   
    end
    
elseif(intruderSpeed>130)
    DR = 6.7*6070;
    %Do not perform scale factor correction once track is established
    %DR scale factor is linearly interpolated between levels
    if(azimuth<=30)
        maxRange = DR*(1-0.16*(azimuth-0)/(30-0)*~prevIsValid);
    elseif(azimuth<=60)
        maxRange = DR*(1-(0.16+0.24*(azimuth-30)/(60-30))*~prevIsValid);   
    elseif(azimuth<=90)
        maxRange = DR*(1-(0.4+0.05*(azimuth-60)/(90-60))*~prevIsValid);   
    elseif(azimuth<=110)
        maxRange = DR*(1-(0.45+0.0*(azimuth-90)/(110-90))*~prevIsValid);   
    end
    
end
    
if(RCPR_Mode)
   rangeValid = range <= maxRange & range >= RCPR_Range_ft;  
else
   rangeValid = range <= maxRange;  
end

== matlab function SC228_TrackedRadarModelUnitTest/SC-228 Sensor Model: Radar (Tracked)/NED2FRD ==
  data: psi_rad input; T output; theta input; phi input
function T = Transform_NED2FRD(psi_rad,theta,phi)
%#codegen

yaw = [ cos(psi_rad) sin(psi_rad) 0;
       -sin(psi_rad) cos(psi_rad) 0;
               0        0 1 ];
           
pitch = [ cos(theta) 0 -sin(theta);
                   0 1           0;
          sin(theta) 0  cos(theta) ];
      
roll = [ 1         0        0;
         0  cos(phi) sin(phi);
         0 -sin(phi) cos(phi) ];
     
T = roll*pitch*yaw;     % transformation FROM geographic coord TO body coord

== matlab function SC228_TrackedRadarModelUnitTest/SC-228 Sensor Model: Radar (Tracked)/Update Rate ==
  data: time input; x_out output; tov_out output; delay input; x input; prev_x input; prev_tov input; update_time input; update_time_out output
function [x_out,tov_out,update_time_out] = fcn(time,delay,x,prev_x,prev_tov,update_time)
%#codegen

if time-update_time>=-0.001 % pass out new output
    update_time_out = time+delay; 
    x_out = x;
    tov_out = time;
else % continue passing out old output
    x_out = prev_x; 
    update_time_out = update_time;
    tov_out = prev_tov;
end
